simulink model "test"  (R2013b)
settings: Solver=ode45  StartTime=0.0  StopTime=10.0  RelTol=1e-3
libraries: xbsIndex_r4 x17, xps_library x1
settings Model: Creator=root  LastModifiedBy=root

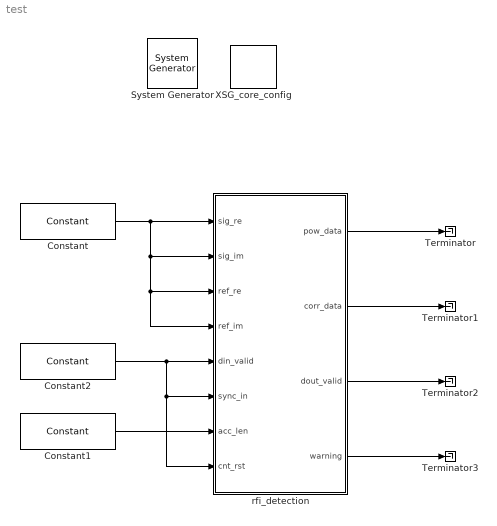
== system test ==
  " System Generator" : xbsIndex_r4/ System Generator  Tag=genX  xilinxfamily=Kintex7  part=xc7k325t  speed=-3  package=fbg676  synthesis_tool=XST  clock_wrapper=Clock Enables  directory=./netlist  proj_type=Project Navigator  Synth_file=XST Defaults  Impl_file=ISE Defaults  testbench=off  simulink_period=1  sysclk_period=10  dcm_input_clock_period=10  incr_netlist=off  trim_vbits=Everywhere in SubSystem  dbl_ovrd=According to Block Masks  core_generation=According to Block Masks  run_coregen=off  deprecated_control=off  eval_field=0  block_type=sysgen
  Constant : xbsIndex_r4/Constant  const=0.5  gui_display_data_type=Fixed-point  arith_type=Signed (2's comp)  n_bits=18  bin_pt=17  preci_type=Single  exp_width=8  frac_width=24  explicit_period=on  period=1  equ=P=C  opselect=C  inp2=PCIN>>17  opr=+  inp1=P  carry=CIN  dbl_ovrd=off  block_type=constant
  Constant1 : xbsIndex_r4/Constant  const=10  gui_display_data_type=Fixed-point  arith_type=Unsigned  n_bits=32  bin_pt=0  preci_type=Single  exp_width=8  frac_width=24  explicit_period=on  period=1  equ=P=C  opselect=C  inp2=PCIN>>17  opr=+  inp1=P  carry=CIN  dbl_ovrd=off  block_type=constant
  Constant2 : xbsIndex_r4/Constant  const=1  gui_display_data_type=Boolean  arith_type=Boolean  n_bits=18  bin_pt=17  preci_type=Single  exp_width=8  frac_width=24  explicit_period=on  period=1  equ=P=C  opselect=C  inp2=PCIN>>17  opr=+  inp1=P  carry=CIN  dbl_ovrd=off  block_type=constant
  Terminator{,1..3} (4 alike) : Terminator
  XSG_core_config : xps_library/XSG_core_config  Tag=xps:xsg  hw_sys=ROACH2:sx475t  clk_src=sys_clk  ROACH_clk_src=sys_clk  ROACH2_clk_src=sys_clk  MKDIG_clk_src=sys_clk  clk_rate=100  sample_period=1  synthesis_tool=XST
  rfi_detection : Subsystem  mask{din_width=18, channel_addr=9, cast_shift=5, cast_delay=1, cast_width=9, cast_point=8, post_mult_delay=0, acc_width=32, post_acc_shift=0, post_acc_width=17, post_acc_point=7, post_acc_delay=2, dout_shift=0, dout_width=18, dout_point=8, debug=1}
      mask prompts: din_width "din width"; channel_addr "channel address"; cast_shift "cast shift"; cast_delay "cast delay"; cast_width "cast width"; cast_point "cast point"; post_mult_delay "post mult delay"; acc_width "acc width"; post_acc_shift "post acc shift"; post_acc_width "post acc width"; post_acc_point "post acc point"; post_acc_delay "post acc delay"; dout_shift "dout shift"; dout_width "dout width"; dout_point "dout point"
  wires:
  Constant/1 -> rfi_detection/2(sig_im), rfi_detection/4(ref_im), rfi_detection/3(ref_re), rfi_detection/1(sig_re)
  Constant1/1 -> rfi_detection/7(acc_len)
  Constant2/1 -> rfi_detection/6(sync_in), rfi_detection/8(cnt_rst), rfi_detection/5(din_valid)
  rfi_detection/1(pow_data) -> Terminator/1
  rfi_detection/2(corr_data) -> Terminator1/1
  rfi_detection/3(dout_valid) -> Terminator2/1
  rfi_detection/4(warning) -> Terminator3/1

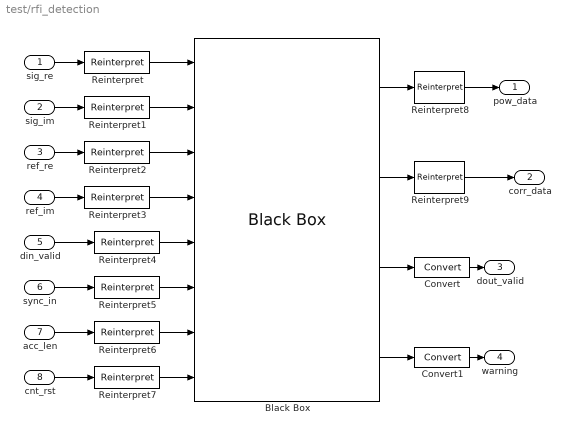
== system test/rfi_detection ==
  sig_re : Inport
  sig_im : Inport  Port=2
  ref_re : Inport  Port=3
  ref_im : Inport  Port=4
  din_valid : Inport  Port=5
  sync_in : Inport  Port=6
  acc_len : Inport  Port=7
  cnt_rst : Inport  Port=8
  Black Box : xbsIndex_r4/Black Box  init_code=rfi_detection_config  sim_method=Inactive  verbose=off  block_type=blackbox2
  Convert : xbsIndex_r4/Convert  gui_display_data_type=Boolean  arith_type=Boolean  n_bits=3  bin_pt=0  float_type=Single  exp_bits=8  fraction_bits=24  quantization=Truncate  overflow=Wrap  en=off  latency=0  dbl_ovrd=off  pipeline=off  block_type=convert
      settings: block_version=11.4
  Convert1 : xbsIndex_r4/Convert  gui_display_data_type=Boolean  arith_type=Boolean  n_bits=3  bin_pt=0  float_type=Single  exp_bits=8  fraction_bits=24  quantization=Truncate  overflow=Wrap  en=off  latency=0  dbl_ovrd=off  pipeline=off  block_type=convert
      settings: block_version=11.4
  Reinterpret{,1..7} (8 alike) : xbsIndex_r4/Reinterpret  force_arith_type=on  arith_type=Unsigned  force_bin_pt=on  bin_pt=0  block_type=reinterpret
  Reinterpret8 : xbsIndex_r4/Reinterpret  force_arith_type=on  arith_type=Unsigned  force_bin_pt=on  bin_pt=dout_point  block_type=reinterpret
  Reinterpret9 : xbsIndex_r4/Reinterpret  force_arith_type=on  arith_type=Unsigned  force_bin_pt=on  bin_pt=dout_point  block_type=reinterpret
  pow_data : Outport
  corr_data : Outport  Port=2
  dout_valid : Outport  Port=3
  warning : Outport  Port=4
  wires:
  din_valid/1 -> Reinterpret4/1
  Black Box/1 -> Reinterpret8/1
  ref_re/1 -> Reinterpret2/1
  sig_re/1 -> Reinterpret/1
  Black Box/4 -> Convert1/1
  ref_im/1 -> Reinterpret3/1
  Black Box/2 -> Reinterpret9/1
  sync_in/1 -> Reinterpret5/1
  cnt_rst/1 -> Reinterpret7/1
  Black Box/3 -> Convert/1
  acc_len/1 -> Reinterpret6/1
  sig_im/1 -> Reinterpret1/1
  Reinterpret/1 -> Black Box/1
  Reinterpret1/1 -> Black Box/2
  Reinterpret2/1 -> Black Box/3
  Reinterpret3/1 -> Black Box/4
  Reinterpret4/1 -> Black Box/5
  Reinterpret5/1 -> Black Box/6
  Reinterpret7/1 -> Black Box/8
  Reinterpret6/1 -> Black Box/7
  Convert/1 -> dout_valid/1
  Convert1/1 -> warning/1
  Reinterpret8/1 -> pow_data/1
  Reinterpret9/1 -> corr_data/1
